simulink model "entryVehicle"  (R2025a)
settings: Solver=ode5  StartTime=startTime  StopTime=stopTime  FixedStep=stepTime  RelTol=1e-3
values from neighbouring files (symbols this model uses):
  alpha_0 = deg2rad(-23.)    [run_entryVehicle.m]
  alpha_T_CD = [0 5 10 15 20 25 30 35 40]    [ApolloDragCoeff.mat]
  alpha_T_CL = [0 5 10 15 20 25 30 35 40]    [ApolloLiftCoeff.mat]
  beta_0 = deg2rad(0.05)    [run_entryVehicle.m]
  CD_T = [1.13 1.305 1.34 1.394 1.445 1.472 1.48 1.468 1.454 1.486 1.51 1.124 ... (99 elements, 11x9)]    [ApolloDragCoeff.mat]
  chi_0 = deg2rad(90)    [run_entryVehicle.m]
  CL_T = [0 0 0 0 0 0 0 0 0 0 0 0.098 ... (99 elements, 11x9)]    [ApolloLiftCoeff.mat]
  d_ref = 3.9    [run_entryVehicle.m]
  gamma_0 = deg2rad(-9.536)    [run_entryVehicle.m]
  H_s = 7050    [run_entryVehicle.m]
  I_xx = 5617.61    [run_entryVehicle.m]
  I_xz = 0    [run_entryVehicle.m]
  I_yy = 4454.62    [run_entryVehicle.m]
  I_zz = 4454.80    (= 4454.8)    [run_entryVehicle.m]
  lambda_0 = deg2rad(0)    [run_entryVehicle.m]
  m_0 = 4976    [run_entryVehicle.m]
  Mach_numbers_CD = [0.9 1.1 1.2 1.35 1.65 2 2.4 3 4 6 10]    [ApolloDragCoeff.mat]
  Mach_numbers_CL = [0.9 1.1 1.2 1.35 1.65 2 2.4 3 4 6 10]    [ApolloLiftCoeff.mat]
  Mars_mu = 3.98319648e14    (= 398319648000000)    [run_entryVehicle.m]
  Mars_radius = 6371e3    (= 6371000)    [run_entryVehicle.m]
  p_0 = deg2rad(0)    [run_entryVehicle.m]
  q_0 = deg2rad(0)    [run_entryVehicle.m]
  r_0 = deg2rad(0)    [run_entryVehicle.m]
  R_0 = 220e3 + Mars_radius    (= 6591000)    [run_entryVehicle.m]
  r_cm = [1.57; 0; -0.137]    [run_entryVehicle.m]
  R_s = 287    [run_entryVehicle.m]
  rho_0 = 1.225    [run_entryVehicle.m]
  S_ref = 12    [run_entryVehicle.m]
  sigma_0 = deg2rad(110.)    [run_entryVehicle.m]
  specific_heat = 1.33    [run_entryVehicle.m]
  stepTime = 0.01    [run_entryVehicle.m]
  tau_0 = deg2rad(0)    [run_entryVehicle.m]
  V_0 = 11e3    (= 11000)    [run_entryVehicle.m]
undefined symbols (not defined in the file or in its folder): A_attitude, acce_bias, acce_S, alpha_T_Cm, alpha_T_Cm_q, B_attitude, Cm_qT, Cm_T, dynamics_constants, K_lat, K_long, lateral_ref, longitudinal_ref, Mach_numbers_Cm, Mach_numbers_Cm_q, my_max, Q0, r0_eci, rateGyro_bias, rateGyro_S, v0_eci
libraries: simulink_extras x32, simulink x3, SignalEditorBlockLib x1
(part 1 of 3)
settings Model: Creator=tester  LastModifiedBy=rafae

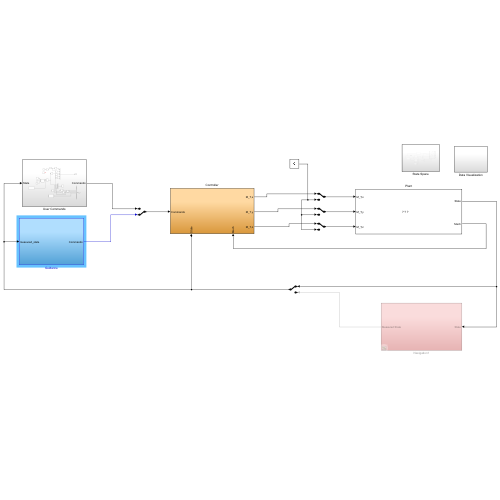
[thumbnail: Simulink's stored preview of the top-level diagram]
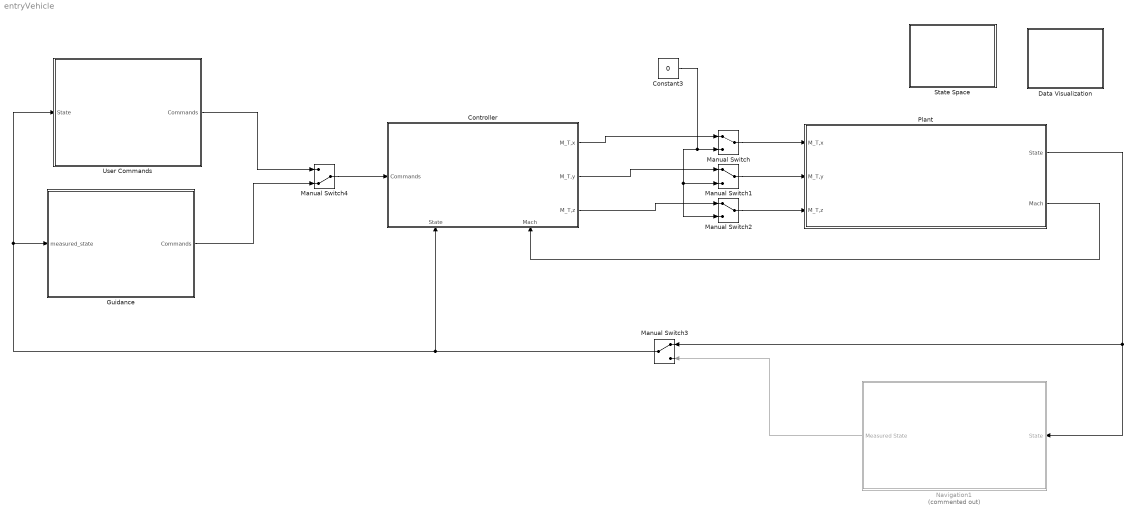
== system entryVehicle ==
  Constant3 : Constant  Value=0
  Controller : Subsystem
      settings: PortSchema="{\"entries\":[{\"content\":{\"sides\":[{\"content\":{\"connectorIds\":[\"In1\"]},\"type\":\"ConnectorPlacement.EquallySpacedRectSide\",\"uuid\":\"6730c763-0db7-4539-af59-842a5691e68e\"},{\"content\":{\"connectorIds\":[\"Out1\",\"Out2\",\"Out3\"],\"side\":\"RIGHT\"},\"type\":\"ConnectorPlacement.EquallySpacedRectSide\",\"uuid\":\"60c274f5-9a0e-4442-9031-a8a2f12bc615\"},{\"content\":{\"side\":\"TOP\"},\"type\":\"ConnectorPlacement.EquallySpacedRectSide\",\"uuid\":\"e1e9f683-9b0b-4096-8ce5-6b557ad43515\"},{\"content\":{\"connectorIds\":[\"In2\",\"In3\"],\"side\":\"BOTTOM\"},\"type\":\"ConnectorPlacement.EquallySpacedRectSide\",\"uuid\":\"b92da982-2d47-4e6b-9095-2c7c1889c431\"}]},\"type\":\"ConnectorPlacement.EquallySpacedConnector\",\"uuid\":\"278978b4-8d2f-4edc-bb2a-9785bc810a53\"}],\"packageUris\":[\"http://schema.mathworks.com/mf0/Connector/R2020b\"],\"version\":\"1.0\"}"
  Data Visualization : Subsystem
  Guidance : Subsystem
  Manual Switch{,1..3} (4 alike) : ManualSwitch
  Manual Switch4 : ManualSwitch  CurrentSetting=0
  Navigation1 : Subsystem  Commented=on
  Plant : Subsystem
      mask Display: image('MSLEntryVehicle.jpg', [0,0,0,0,100,90]);
  State Space : Subsystem
  User Commands : Subsystem
  wires:
  Controller/1(M_T,x) -> Manual Switch/1
  Manual Switch/1 -> Plant/1(M_T,x)
  Manual Switch2/1 -> Plant/3(M_T,z)
  Manual Switch1/1 -> Plant/2(M_T,y)
  Controller/2(M_T,y) -> Manual Switch1/1
  Controller/3(M_T,z) -> Manual Switch2/1
  Constant3/1 -> Manual Switch1/2, Manual Switch2/2, Manual Switch/2
  Plant/1(State) -> Navigation1/1(State), Manual Switch3/1
  Plant/2(Mach) -> Controller/3(Mach)
  User Commands/1(Commands) -> Manual Switch4/1
  Guidance/1(Commands) -> Manual Switch4/2
  Manual Switch4/1 -> Controller/1(Commands)
  Navigation1/1(Measured State) -> Manual Switch3/2
  Manual Switch3/1 -> Controller/2(State), User Commands/1(State), Guidance/1(measured_state)

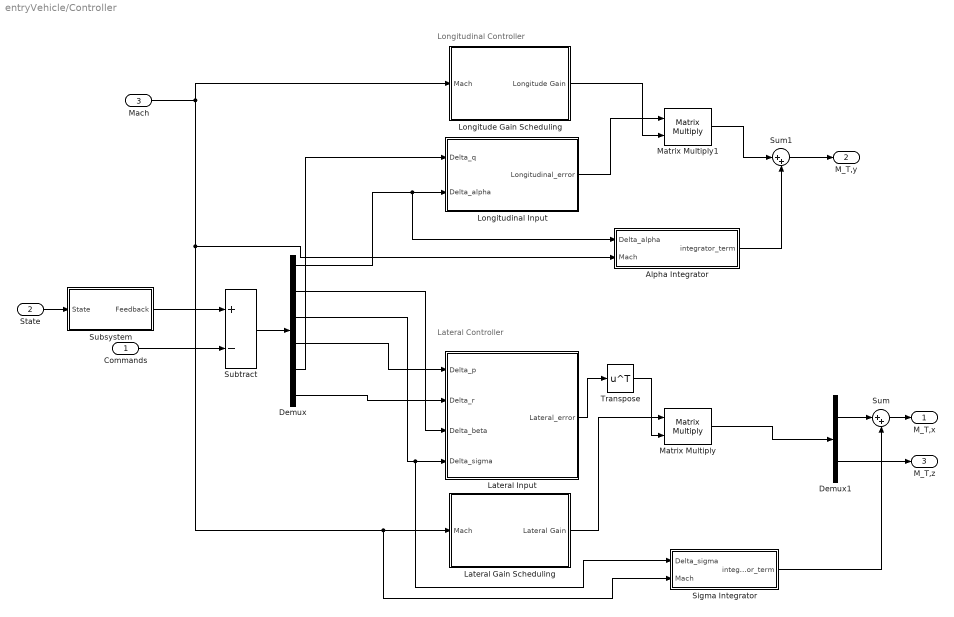
== system entryVehicle/Controller ==
  note: Lateral Controller
  note: Longitudinal Controller
  Commands : Inport
  State : Inport  Port=2
  Mach : Inport  Port=3
  Alpha Integrator : Subsystem
  Demux : Demux  Outputs=6
  Demux1 : Demux  Outputs=2
  Lateral Gain Scheduling : Subsystem
  Lateral Input : Subsystem
  Longitude Gain Scheduling : Subsystem
  Longitudinal Input : Subsystem
  Matrix Multiply : Product  Multiplication=Matrix(*)
  Matrix Multiply1 : Product  Multiplication=Matrix(*)
  Sigma Integrator : Subsystem
  Subsystem : Subsystem
  Subtract : Sum  Inputs=+-
  Sum : Sum  Inputs=|++
  Sum1 : Sum  Inputs=|++
  Transpose : Math  Operator=transpose
  M_T,x : Outport
  M_T,y : Outport  Port=2
  M_T,z : Outport  Port=3
  wires:
  State/1 -> Subsystem/1(State)
  Demux/1 -> Alpha Integrator/1(Delta_alpha), Longitudinal Input/2(Delta_alpha)
  Demux/5 -> Longitudinal Input/1(Delta_q)
  Demux/2 -> Lateral Input/3(Delta_beta)
  Demux/3 -> Lateral Input/4(Delta_sigma), Sigma Integrator/1(Delta_sigma)
  Demux/4 -> Lateral Input/1(Delta_p)
  Demux/6 -> Lateral Input/2(Delta_r)
  Commands/1 -> Subtract/2
  Subtract/1 -> Demux/1
  Subsystem/1(Feedback) -> Subtract/1
  Mach/1 -> Longitude Gain Scheduling/1(Mach), Alpha Integrator/2(Mach), Sigma Integrator/2(Mach), Lateral Gain Scheduling/1(Mach)
  Longitudinal Input/1(Longitudinal_error) -> Matrix Multiply1/1
  Longitude Gain Scheduling/1(Longitude Gain) -> Matrix Multiply1/2
  Matrix Multiply/1 -> Demux1/1
  Demux1/1 -> Sum/1
  Sum/1 -> M_T,x/1
  Matrix Multiply1/1 -> Sum1/1
  Sum1/1 -> M_T,y/1
  Demux1/2 -> M_T,z/1
  Lateral Gain Scheduling/1(Lateral Gain) -> Matrix Multiply/1
  Lateral Input/1(Lateral_error) -> Transpose/1
  Transpose/1 -> Matrix Multiply/2
  Alpha Integrator/1(integrator_term) -> Sum1/2
  Sigma Integrator/1(integrator_term) -> Sum/2

== system entryVehicle/Data Visualization ==

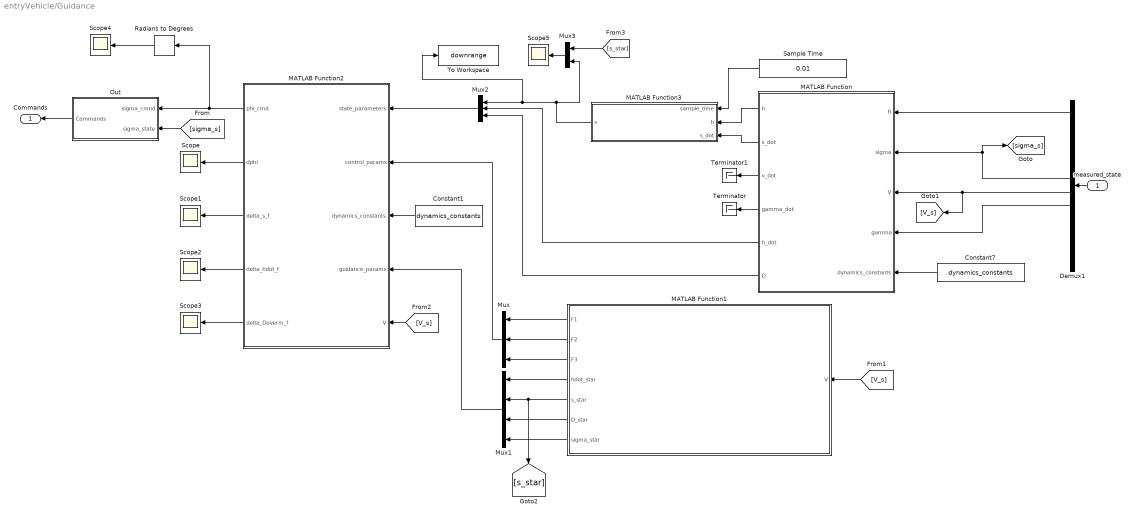
== system entryVehicle/Guidance ==
  measured_state : Inport
  Constant1 : Constant  Value=dynamics_constants
  Constant7 : Constant  Value=dynamics_constants
  Demux1 : Demux  Outputs=12
  MATLAB Function : MATLAB Function  TreatAsAtomicUnit=on
  MATLAB Function1 : MATLAB Function  TreatAsAtomicUnit=on
  MATLAB Function2 : MATLAB Function  TreatAsAtomicUnit=on  SystemSampleTime=1
  MATLAB Function3 : MATLAB Function  TreatAsAtomicUnit=on  SystemSampleTime=0.01
  Mux : Mux  Inputs=3
  Mux1 : Mux
  Mux2 : Mux  Inputs=3
  Mux3 : Mux  Inputs=2
  Out : Subsystem
  Radians to Degrees : simulink_extras/Transformations/Radians to Degrees
  Sample Time : Constant  Value=0.01
  Scope{,1..5} (6 alike) : Scope
      Scope settings: ActiveDisplayYMinimum=-0.02182  ActiveDisplayYMaximum=0.19635
      Scope1 settings: ActiveDisplayYMinimum=-5846.34757  ActiveDisplayYMaximum=52617.12815  DataLoggingVariableName=ScopeData2
      Scope2 settings: ActiveDisplayYMinimum=-1.55731  ActiveDisplayYMaximum=13.66679  DataLoggingVariableName=ScopeData3
      Scope3 settings: ActiveDisplayYMinimum=-781.36553  ActiveDisplayYMaximum=1579.10132  DataLoggingVariableName=ScopeData4
      Scope4 settings: ActiveDisplayYMinimum=4.375  ActiveDisplayYMaximum=110.625
      Scope5 settings: ActiveDisplayYMinimum=-224179.17494  ActiveDisplayYMaximum=2.01869737437E+6
  Terminator : Terminator
  Terminator1 : Terminator
  To Workspace : ToWorkspace  VariableName=downrange  SaveFormat=Structure With Time  SampleTime=-1
  Commands : Outport
  wires:
  measured_state/1 -> Demux1/1
  MATLAB Function/4(gamma_dot) -> Terminator/1
  Out/1(Commands) -> Commands/1
  Constant7/1 -> MATLAB Function/5(dynamics_constants)
  Demux1/1 -> MATLAB Function/1(R)
  Demux1/6 -> MATLAB Function/2(sigma), [sigma_s]
  Demux1/7 -> [V_s], MATLAB Function/3(V)
  Demux1/8 -> MATLAB Function/4(gamma)
  MATLAB Function/3(v_dot) -> Terminator1/1
  MATLAB Function/1(h) -> MATLAB Function3/2(h)
  MATLAB Function/2(s_dot) -> MATLAB Function3/3(s_dot)
  Sample Time/1 -> MATLAB Function3/1(sample_time)
  MATLAB Function1/1(F1) -> Mux/1
  MATLAB Function1/2(F2) -> Mux/2
  MATLAB Function1/3(F3) -> Mux/3
  MATLAB Function1/4(hdot_star) -> Mux1/1
  MATLAB Function1/5(s_star) -> Mux1/2, [s_star]
  MATLAB Function1/6(D_star) -> Mux1/3
  MATLAB Function1/7(sigma_star) -> Mux1/4
  MATLAB Function3/1(s) -> Mux3/2, Mux2/1, To Workspace/1
  MATLAB Function/5(h_dot) -> Mux2/2
  MATLAB Function/6(D) -> Mux2/3
  Mux2/1 -> MATLAB Function2/1(state_parameters)
  Mux/1 -> MATLAB Function2/2(control_params)
  Mux1/1 -> MATLAB Function2/4(guidance_params)
  Constant1/1 -> MATLAB Function2/3(dynamics_constants)
  MATLAB Function2/1(phi_cmd) -> Radians to Degrees/1, Out/1(sigma_cmnd)
  MATLAB Function2/2(dphi) -> Scope/1
  MATLAB Function2/3(delta_s_f) -> Scope1/1
  MATLAB Function2/4(delta_hdot_f) -> Scope2/1
  MATLAB Function2/5(delta_Doverm_f) -> Scope3/1
  Radians to Degrees/1 -> Scope4/1
  [sigma_s] -> Out/2(sigma_state)
  [V_s] -> MATLAB Function1/1(V)
  [V_s] -> MATLAB Function2/5(V)
  [s_star] -> Mux3/1
  Mux3/1 -> Scope5/1

== system entryVehicle/Navigation1 ==
  State : Inport
  Abs : Abs  SaturateOnIntegerOverflow=off
  Demux : Demux  Outputs=12
  Demux1 : Demux  Outputs=12
  Derivative : Derivative
  ECI State Propagation : Subsystem
  ECI State to State : Subsystem
  IMU Sensor : Subsystem
  MATLAB Function : MATLAB Function  TreatAsAtomicUnit=on
  Mux2 : Mux  Inputs=2
  Mux5 : Mux  Inputs=2
  Scope2 : Scope
      settings: ActiveDisplayYMinimum=-14.28055  ActiveDisplayYMaximum=128.52494  DataLoggingVariableName=ScopeData3
  Scope4 : Scope
      settings: ActiveDisplayYMinimum=-1.3626  ActiveDisplayYMaximum=0.15263  DataLoggingVariableName=ScopeData7
  State to Body (acce minus gravity) : Subsystem
  Measured State : Outport
  wires:
  State/1 -> Demux/1, State to Body (acce minus gravity)/1(state)
  ECI State to State/1(meas_state) -> Demux1/1, Measured State/1
  State to Body (acce minus gravity)/1(acce_body) -> IMU Sensor/1(acce_body), MATLAB Function/1(u)
  State to Body (acce minus gravity)/2(omega_body) -> IMU Sensor/2(omega_body)
  IMU Sensor/1(a_meas) -> ECI State Propagation/1(a_meas)
  IMU Sensor/2(omega_meas) -> ECI State Propagation/2(omega_meas)
  ECI State Propagation/1(meas_state_ECI) -> ECI State to State/1(meas_state_ECI)
  Abs/1 -> Mux2/1
  MATLAB Function/1(y) -> Mux2/2
  Mux2/1 -> Scope2/1
  Derivative/1 -> Abs/1
  Demux1/8 -> Mux5/2
  Mux5/1 -> Scope4/1
  Demux/7 -> Derivative/1
  State to Body (acce minus gravity)/3(Qtrue) -> ECI State Propagation/3(Q_true)
  Demux/8 -> Mux5/1

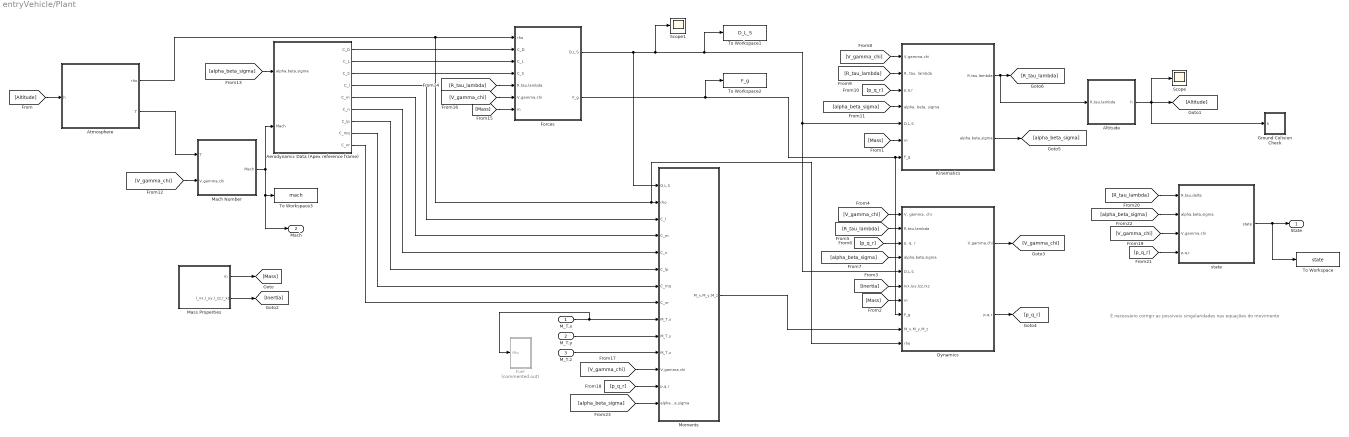
== system entryVehicle/Plant ==
  note: É necessário corrigir as possíveis singularidades nas equações do movimento
  M_T,x : Inport
  M_T,y : Inport  Port=2
  M_T,z : Inport  Port=3
  Aerodynamic Data (Apex reference frame) : Subsystem
  Altitude : Subsystem
  Atmosphere : Subsystem
  Dynamics : Subsystem
  Forces : Subsystem
  Fuel : Subsystem  Commented=on
  Ground Colision Check : Subsystem
  Kinematics : Subsystem
  Mach Number : Subsystem
  Mass Properties : Subsystem
  Moments : Subsystem
  Scope : Scope
      settings: ActiveDisplayYMinimum=-27500.49137  ActiveDisplayYMaximum=247500.0546  YLabel=m  DataLoggingVariableName=ScopeData7
  Scope1 : Scope
      settings: ActiveDisplayYMinimum=-224326.20631  ActiveDisplayYMaximum=477184.42934  DataLoggingVariableName=ScopeData2
  To Workspace : ToWorkspace  VariableName=state  SaveFormat=Structure With Time  SampleTime=-1
  To Workspace1 : ToWorkspace  VariableName=D_L_S  SaveFormat=Structure With Time  SampleTime=-1
  To Workspace2 : ToWorkspace  VariableName=F_g  SaveFormat=Structure With Time  SampleTime=-1
  To Workspace3 : ToWorkspace  VariableName=mach  SaveFormat=Structure With Time  SampleTime=-1
  state : Subsystem
  State : Outport
  Mach : Outport  Port=2
  wires:
  M_T,x/1 -> Fuel/1(Mtx), Moments/9(M_T,x)
  M_T,y/1 -> Moments/10(M_T,y)
  M_T,z/1 -> Moments/11(M_T,z)
  Aerodynamic Data (Apex reference frame)/6(C_n) -> Moments/5(C_n)
  Aerodynamic Data (Apex reference frame)/5(C_m) -> Moments/4(C_m)
  Aerodynamic Data (Apex reference frame)/4(C_l) -> Moments/3(C_l)
  Altitude/1(h) -> [Altitude], Scope/1, Ground Colision Check/1(h)
  [Altitude] -> Atmosphere/1(h)
  Mass Properties/1(m) -> [Mass]
  [Mass] -> Kinematics/6(m)
  Mass Properties/2(I_xx,I_yy,I_zz,I_xz) -> [Inertia]
  Forces/2(F_g) -> To Workspace2/1, Dynamics/8(F_g), Kinematics/7(F_g)
  [Mass] -> Dynamics/7(m)
  [Inertia] -> Dynamics/6(Ixx,Iyy,Izz,Ixz)
  Forces/1(D,L,S) -> Scope1/1, To Workspace1/1, Dynamics/5(D,L,S), Kinematics/5(D,L,S), Moments/1(D,L,S)
  Moments/1(M_x,M_y,M_z) -> Dynamics/9(M_x,M_y,M_z)
  Dynamics/2(p,q,r) -> [p_q_r]
  Dynamics/1(V,gamma,chi) -> [V_gamma_chi]
  Kinematics/2(alpha,beta,sigma) -> [alpha_beta_sigma]
  [V_gamma_chi] -> Dynamics/1("V, gamma, chi")
  [R_tau_lambda] -> Dynamics/2(R,tau,lambda)
  Kinematics/1(R,tau,lambda) -> [R_tau_lambda], Altitude/1(R,tau,lambda)
  [p_q_r] -> Dynamics/3("p, q, r")
  [alpha_beta_sigma] -> Dynamics/4(alpha,beta,sigma)
  [V_gamma_chi] -> Kinematics/1(V,gamma,chi)
  [R_tau_lambda] -> Kinematics/2("R, tau, lambda")
  [p_q_r] -> Kinematics/3(p,q,r)
  [alpha_beta_sigma] -> Kinematics/4("alpha, beta, sigma")
  Mach Number/1(Mach) -> To Workspace3/1, Mach/1, Aerodynamic Data (Apex reference frame)/2(Mach)
  [V_gamma_chi] -> Mach Number/2(V,gamma,chi)
  Atmosphere/1(rho) -> Dynamics/10(rho), Moments/2(rho), Forces/1(rho)
  [alpha_beta_sigma] -> Aerodynamic Data (Apex reference frame)/1(alpha,beta,sigma)
  [R_tau_lambda] -> Forces/5(R,tau,lambda)
  [Mass] -> Forces/7(m)
  [V_gamma_chi] -> Forces/6(V,gamma,chi)
  [V_gamma_chi] -> Moments/12(V,gamma,chi)
  Atmosphere/2(T) -> Mach Number/1(T)
  Aerodynamic Data (Apex reference frame)/1(C_D) -> Forces/2(C_D)
  Aerodynamic Data (Apex reference frame)/2(C_L) -> Forces/3(C_L)
  Aerodynamic Data (Apex reference frame)/3(C_S) -> Forces/4(C_S)
  [p_q_r] -> Moments/13(p,q,r)
  Aerodynamic Data (Apex reference frame)/9(C_nr) -> Moments/8(C_nr)
  Aerodynamic Data (Apex reference frame)/8(C_mq) -> Moments/7(C_mq)
  Aerodynamic Data (Apex reference frame)/7(C_lp) -> Moments/6(C_lp)
  [V_gamma_chi] -> state/3(V,gamma,chi)
  [R_tau_lambda] -> state/1(R,tau,delta)
  [p_q_r] -> state/4(p,q,r)
  [alpha_beta_sigma] -> state/2(alpha,beta,sigma)
  state/1(state) -> To Workspace/1, State/1
  [alpha_beta_sigma] -> Moments/14(alpha,beta,sigma)

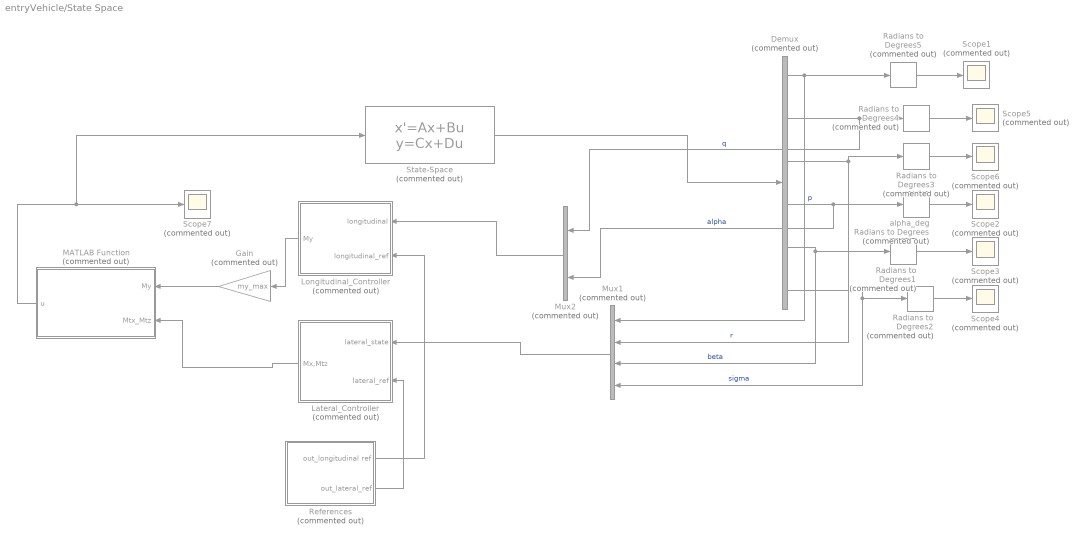
== system entryVehicle/State Space ==
  Demux : Demux  Commented=on  Outputs=6
  Gain : Gain  Commented=on  Gain=my_max
  Lateral_Controller : Subsystem  Commented=on
  Longitudinal_Controller : Subsystem  Commented=on
  MATLAB Function : MATLAB Function  Commented=on  TreatAsAtomicUnit=on
  Mux1 : Mux  Commented=on
  Mux2 : Mux  Commented=on  Inputs=2
  Radians to Degrees{1..5} (5 alike) : simulink_extras/Transformations/Radians to Degrees  Commented=on
  References : Subsystem  Commented=on
  Scope{1..7} (7 alike) : Scope  Commented=on
      Scope1 settings: ActiveDisplayYMinimum=-1.19941  ActiveDisplayYMaximum=0.17016
      Scope2 settings: ActiveDisplayYMinimum=-1.81589  ActiveDisplayYMaximum=2.88928  DataLoggingVariableName=ScopeData2
      Scope3 settings: ActiveDisplayYMinimum=-0.00061  ActiveDisplayYMaximum=0.00135
      Scope4 settings: ActiveDisplayYMinimum=-3.22061  ActiveDisplayYMaximum=28.98549  DataLoggingVariableName=ScopeData2
      Scope5 settings: ActiveDisplayYMinimum=-44.27214  ActiveDisplayYMaximum=39.05439  DataLoggingVariableName=ScopeData3
      Scope6 settings: ActiveDisplayYMinimum=-0.06363  ActiveDisplayYMaximum=0.53909  DataLoggingVariableName=ScopeData4
      Scope7 settings: ActiveDisplayYMinimum=-66691.93639  ActiveDisplayYMaximum=44857.66818  DataLoggingVariableName=ScopeData5
  State-Space : StateSpace  Commented=on  A=A_attitude  B=B_attitude  C=eye(6)  D=zeros(6,3)  InitialCondition=[0; 0; 0; -0.101; 0; 0]
  alpha_deg : simulink_extras/Transformations/Radians to Degrees  Commented=on
  wires:
  Radians to Degrees1/1 -> Scope3/1
  MATLAB Function/1(u) -> Scope7/1, State-Space/1
  Demux/4 -> alpha_deg/1, Mux2/2  "alpha"
  Radians to Degrees2/1 -> Scope4/1
  Lateral_Controller/1(Mx,Mtz) -> MATLAB Function/2(Mtx_Mtz)
  Demux/1 -> Mux1/1, Radians to Degrees5/1  "p"
  Longitudinal_Controller/1(My) -> Gain/1
  Demux/3 -> Mux1/2, Radians to Degrees3/1  "r"
  Demux/2 -> Mux2/1, Radians to Degrees4/1  "q"
  Demux/5 -> Mux1/3, Radians to Degrees1/1  "beta"
  Radians to Degrees3/1 -> Scope6/1
  Radians to Degrees5/1 -> Scope1/1
  Radians to Degrees4/1 -> Scope5/1
  Demux/6 -> Mux1/4, Radians to Degrees2/1  "sigma"
  State-Space/1 -> Demux/1
  alpha_deg/1 -> Scope2/1
  References/1(out_longitudinal ref) -> Longitudinal_Controller/2(longitudinal_ref)
  Mux1/1 -> Lateral_Controller/1(lateral_state)
  References/2(out_lateral_ref) -> Lateral_Controller/2(lateral_ref)
  Gain/1 -> MATLAB Function/1(My)
  Mux2/1 -> Longitudinal_Controller/1(longitudinal)

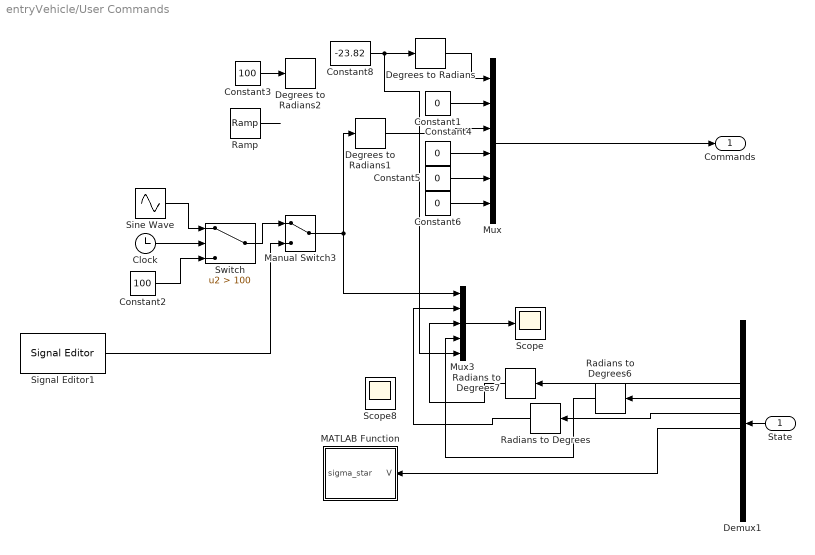
== system entryVehicle/User Commands ==
  State : Inport
  Clock : Clock
  Constant{1,4..6} (4 alike) : Constant  Value=0
  Constant2 : Constant  Value=100
  Constant3 : Constant  Value=100
  Constant8 : Constant  Value=-23.82
  Degrees to Radians : simulink_extras/Transformations/Degrees to Radians
  Degrees to Radians1 : simulink_extras/Transformations/Degrees to Radians
  Degrees to Radians2 : simulink_extras/Transformations/Degrees to Radians
  Demux1 : Demux  Outputs=12
  MATLAB Function : MATLAB Function  TreatAsAtomicUnit=on
  Manual Switch3 : ManualSwitch
  Mux : Mux  Inputs=6
  Mux3 : Mux  Inputs=5
  Radians to Degrees : simulink_extras/Transformations/Radians to Degrees
  Radians to Degrees6 : simulink_extras/Transformations/Radians to Degrees
  Radians to Degrees7 : simulink_extras/Transformations/Radians to Degrees
  Ramp : simulink/Sources/Ramp  slope=1  start=100  InitialOutput=70
  Scope : Scope
      settings: ActiveDisplayYMinimum=-42.06517  ActiveDisplayYMaximum=138.41018
  Scope8 : Scope
      settings: ActiveDisplayYMinimum=-1  ActiveDisplayYMaximum=1
  Signal Editor1 : SignalEditorBlockLib/Signal Editor  FileName=sigma_ref_dataset.mat  ActiveScenario=signalDataset  ActiveSignal=sigma_ref  IsBus=off  OutputBusObjectStr=Bus: BusObject  SampleTime=0  Interpolate=off  ZeroCross=off  OutputAfterFinalValue=Setting to zero  Unit=inherit  PreserveSignalName=on  ApplySigPropsToAllScenarios=on  ApplySigPropsToAllSignals=off
  Sine Wave : Sin  Amplitude=20  Bias=100  Frequency=0.05  Phase=1.2  SampleTime=0
  Switch : Switch  Criteria=u2 > Threshold  Threshold=100  SaturateOnIntegerOverflow=off  InputSameDT=off
  Commands : Outport
  wires:
  Radians to Degrees/1 -> Mux3/2
  Constant5/1 -> Mux/5
  Ramp/1 -> ?
  State/1 -> Demux1/1
  Constant4/1 -> Mux/4
  Sine Wave/1 -> Switch/1
  Constant6/1 -> Mux/6
  Demux1/5 -> Radians to Degrees6/1
  Radians to Degrees7/1 -> Mux3/3
  Constant2/1 -> Switch/3
  Degrees to Radians/1 -> Mux/1
  Mux/1 -> Commands/1
  Constant8/1 -> Mux3/5, Degrees to Radians/1
  Switch/1 -> Manual Switch3/1
  Manual Switch3/1 -> Mux3/1, Degrees to Radians1/1
  Mux3/1 -> Scope/1
  Demux1/4 -> Radians to Degrees7/1
  Demux1/6 -> Radians to Degrees/1
  Clock/1 -> Switch/2
  Constant1/1 -> Mux/2
  Radians to Degrees6/1 -> Mux3/4
  Demux1/7 -> MATLAB Function/1(V)
  Constant3/1 -> Degrees to Radians2/1
  Degrees to Radians1/1 -> Mux/3
  Signal Editor1/1 -> Manual Switch3/2

== system entryVehicle/Controller/Alpha Integrator ==
  Delta_alpha : Inport
  Mach : Inport  Port=2
  Gain1 : Gain  Gain=-1
  Gain2 : Gain  Gain=-1/100
  Integrator : Integrator
  MATLAB Function : MATLAB Function  TreatAsAtomicUnit=on
  Product : Product
  Scope : Scope
      settings: ActiveDisplayYMinimum=-61830.77216  ActiveDisplayYMaximum=555371.2989
  integrator_term : Outport
  wires:
  Delta_alpha/1 -> Integrator/1
  Mach/1 -> MATLAB Function/1(Mach)
  Integrator/1 -> Product/1
  MATLAB Function/1(K_integrator_alpha) -> Gain2/1, Scope/1
  Product/1 -> integrator_term/1
  Gain2/1 -> Product/2

== system entryVehicle/Controller/Lateral Gain Scheduling ==
  Mach : Inport
  Gain : Gain  Gain=-1
  MATLAB Function : MATLAB Function  TreatAsAtomicUnit=on
  Lateral Gain : Outport
  wires:
  Mach/1 -> MATLAB Function/1(Mach)
  Gain/1 -> Lateral Gain/1
  MATLAB Function/1(K_lat) -> Gain/1

== system entryVehicle/Controller/Lateral Input ==
  Delta_p : Inport
  Delta_r : Inport  Port=2
  Delta_beta : Inport  Port=3
  Delta_sigma : Inport  Port=4
  Mux : Mux
  Transpose : Math  Operator=transpose
  Lateral_error : Outport
  wires:
  Mux/1 -> Transpose/1
  Delta_r/1 -> Mux/2
  Delta_beta/1 -> Mux/3
  Transpose/1 -> Lateral_error/1
  Delta_p/1 -> Mux/1
  Delta_sigma/1 -> Mux/4

== system entryVehicle/Controller/Longitude Gain Scheduling ==
  Mach : Inport
  Gain : Gain  Gain=-1
  MATLAB Function : MATLAB Function  TreatAsAtomicUnit=on
  Longitude Gain : Outport
  wires:
  Mach/1 -> MATLAB Function/1(Mach)
  MATLAB Function/1(K_long) -> Gain/1
  Gain/1 -> Longitude Gain/1

== system entryVehicle/Controller/Longitudinal Input ==
  Delta_q : Inport
  Delta_alpha : Inport  Port=2
  Mux : Mux  Inputs=2
  Transpose1 : Math  Operator=transpose
  Longitudinal_error : Outport
  wires:
  Delta_q/1 -> Mux/1
  Delta_alpha/1 -> Mux/2
  Mux/1 -> Transpose1/1
  Transpose1/1 -> Longitudinal_error/1

== system entryVehicle/Controller/Sigma Integrator ==
  Delta_sigma : Inport
  Mach : Inport  Port=2
  Gain1 : Gain  Gain=1/100
  Gain2 : Gain
  Integrator : Integrator
  MATLAB Function : MATLAB Function  TreatAsAtomicUnit=on
  Product : Product
  Scope : Scope
      settings: ActiveDisplayYMinimum=-61830.77216  ActiveDisplayYMaximum=555371.2989
  integrator_term : Outport
  wires:
  Delta_sigma/1 -> Integrator/1
  Mach/1 -> MATLAB Function/1(Mach)
  Integrator/1 -> Product/1
  MATLAB Function/1(K_integrator_sigma) -> Gain1/1, Scope/1
  Product/1 -> integrator_term/1
  Gain1/1 -> Product/2

== system entryVehicle/Controller/Subsystem ==
  State : Inport
  Demux : Demux  Outputs=12
  Mux : Mux  Inputs=6
  Feedback : Outport
  wires:
  State/1 -> Demux/1
  Mux/1 -> Feedback/1
  Demux/4 -> Mux/1  "alpha"
  Demux/5 -> Mux/2  "beta"
  Demux/6 -> Mux/3  "sigma"
  Demux/10 -> Mux/4  "p"
  Demux/12 -> Mux/6  "r"
  Demux/11 -> Mux/5  "q"

== system entryVehicle/Guidance/Out ==
  sigma_cmnd : Inport
  sigma_state : Inport  Port=2
  Constant{7,9..11} (4 alike) : Constant  Value=0
  Constant8 : Constant  Value=-23.82
  Degrees to Radians : simulink_extras/Transformations/Degrees to Radians
  Mux : Mux  Inputs=2
  Mux3 : Mux  Inputs=6
  Radians to Degrees : simulink_extras/Transformations/Radians to Degrees
  Scope : Scope
      settings: ActiveDisplayYMinimum=1.32812  ActiveDisplayYMaximum=136.03251  DataLoggingVariableName=ScopeData3
  Commands : Outport
  wires:
  Constant7/1 -> Mux3/2
  Constant11/1 -> Mux3/6
  Mux3/1 -> Commands/1
  Constant8/1 -> Degrees to Radians/1
  Constant10/1 -> Mux3/5
  Degrees to Radians/1 -> Mux3/1
  Constant9/1 -> Mux3/4
  sigma_cmnd/1 -> Mux/1, Mux3/3
  sigma_state/1 -> Mux/2
  Mux/1 -> Radians to Degrees/1
  Radians to Degrees/1 -> Scope/1

== system entryVehicle/Navigation1/ECI State Propagation ==
  note: Inertial Position Propagation
  note: Inertial Velocity Propagation
  note: Intertial Attitude Propagation
  a_meas : Inport
  omega_meas : Inport  Port=2
  Q_true : Inport  Port=3
  Constant : Constant  Value=Mars_mu
  Integrator3 : Integrator  InitialCondition=Q0
  Integrator4 : Integrator  InitialCondition=v0_eci
  Integrator5 : Integrator  InitialCondition=r0_eci
  MATLAB Function : MATLAB Function  TreatAsAtomicUnit=on
  MATLAB Function1 : MATLAB Function  TreatAsAtomicUnit=on
  MATLAB Function2 : MATLAB Function  TreatAsAtomicUnit=on
  MATLAB Function3 : MATLAB Function  TreatAsAtomicUnit=on
  Mux : Mux
  Product1 : Product  Multiplication=Matrix(*)
  Scope : Scope
      settings: DataLoggingVariableName=ScopeData10
  Sum1 : Sum  Inputs=|++
  meas_state_ECI : Outport
  wires:
  omega_meas/1 -> MATLAB Function2/2(omega), Mux/4  "omega_meas"
  Integrator3/1 -> MATLAB Function/1(Q_in)
  MATLAB Function1/1(TIC) -> Product1/1
  a_meas/1 -> Product1/2
  Product1/1 -> Sum1/1
  Sum1/1 -> Integrator4/1
  Integrator4/1 -> Mux/2, Integrator5/1  "v_meas_ECI"
  Integrator5/1 -> MATLAB Function3/1(r_ECI), Mux/1  "r_meas_ECI"
  Mux/1 -> meas_state_ECI/1
  MATLAB Function3/1(g_vec_ECI) -> Scope/1, Sum1/2
  Constant/1 -> MATLAB Function3/2(mu)
  MATLAB Function2/1(Q_dot) -> Integrator3/1
  MATLAB Function/1(Q_out) -> MATLAB Function2/1(Q)  "Q_meas_ECI"
  Q_true/1 -> Mux/3, MATLAB Function1/1(Q)

== system entryVehicle/Navigation1/ECI State to State ==
  meas_state_ECI : Inport
  V_gamma_chi : Inport  Port=2
  R_tau_delta : Inport  Port=3
  Demux : Demux  Outputs=13
  MATLAB Function : MATLAB Function  TreatAsAtomicUnit=on
  MATLAB Function1 : MATLAB Function  TreatAsAtomicUnit=on
  MATLAB Function3 : MATLAB Function  TreatAsAtomicUnit=on
  Mux : Mux  Inputs=3
  Mux1 : Mux  Inputs=3
  Mux2 : Mux
  Mux3 : Mux  Inputs=3
  Mux4 : Mux
  meas_state : Outport
  wires:
  meas_state_ECI/1 -> Demux/1
  Demux/2 -> Mux/2  "r_y"
  Demux/6 -> Mux1/3  "v_z"
  Demux/5 -> Mux1/2  "v_y"
  Demux/3 -> Mux/3  "r_z"
  Demux/1 -> Mux/1  "r_x"
  Demux/4 -> Mux1/1  "v_x"
  Demux/7 -> Mux2/1  "q1"
  Demux/8 -> Mux2/2  "q2"
  Demux/9 -> Mux2/3  "q3"
  Demux/10 -> Mux2/4  "q4"
  Mux/1 -> MATLAB Function/1(r_ECI)  "r_ECI"
  Mux1/1 -> MATLAB Function1/1(v_ECI)  "v_ECI"
  Mux2/1 -> MATLAB Function3/1(Q)  "Q"
  MATLAB Function1/1(V_gamma_chi) -> MATLAB Function3/2(V_gamma_chi), Mux4/3
  MATLAB Function/1(R_tau_delta) -> MATLAB Function3/3(R_tau_delta), MATLAB Function1/2(R_tau_delta), Mux4/1
  Demux/13 -> Mux3/3  "r"
  Demux/11 -> Mux3/1  "p"
  Demux/12 -> Mux3/2  "q"
  Mux4/1 -> meas_state/1
  MATLAB Function3/1(alpha_beta_sigma) -> Mux4/2
  Mux3/1 -> Mux4/4  "p_q_r"

== system entryVehicle/Navigation1/IMU Sensor ==
  note: Rate Gyroscopes
  note: Accelerometers
  acce_body : Inport
  omega_body : Inport  Port=2
  Accelerometer Sensor Noise : simulink/Sources/Band-Limited White Noise  Cov=[0.1]  Ts=stepTime  seed=[23341]
  Constant : Constant  Value=acce_bias
  Constant1 : Constant  Value=acce_S
  Constant2 : Constant  Value=rateGyro_bias
  Constant3 : Constant  Value=rateGyro_S
  Constant4 : Constant  Value=0
  Constant5 : Constant  Value=0
  MATLAB Function : MATLAB Function  TreatAsAtomicUnit=on
  MATLAB Function1 : MATLAB Function  TreatAsAtomicUnit=on
  Manual Switch : ManualSwitch
  Manual Switch1 : ManualSwitch
  Rate Gyro Sensor Noise : simulink/Sources/Band-Limited White Noise  Cov=[0.1]  Ts=stepTime  seed=[23341]
  Sum : Sum  Inputs=|++
  Sum1 : Sum  Inputs=|++
  a_meas : Outport
  omega_meas : Outport  Port=2
  wires:
  Constant/1 -> MATLAB Function/2(b_a)
  acce_body/1 -> MATLAB Function/1(a_body)
  Constant1/1 -> MATLAB Function/3(S_a)
  omega_body/1 -> MATLAB Function1/1(omega_true)
  Constant3/1 -> MATLAB Function1/3(S_omega)
  Constant2/1 -> MATLAB Function1/2(b_gyro)
  MATLAB Function/1(a_measured) -> Sum/1
  Sum/1 -> a_meas/1
  MATLAB Function1/1(omega_measured) -> Sum1/1
  Sum1/1 -> omega_meas/1
  Manual Switch/1 -> Sum/2
  Accelerometer Sensor Noise/1 -> Manual Switch/2
  Constant4/1 -> Manual Switch/1
  Constant5/1 -> Manual Switch1/1
  Manual Switch1/1 -> Sum1/2
  Rate Gyro Sensor Noise/1 -> Manual Switch1/2

== system entryVehicle/Navigation1/State to Body (acce minus gravity) ==
  state : Inport
  Constant : Constant  Value=Mars_mu
  Demux2 : Demux  Outputs=12
  Derivative1 : Derivative
  MATLAB Function : MATLAB Function  TreatAsAtomicUnit=on
  MATLAB Function1 : MATLAB Function  TreatAsAtomicUnit=on
  MATLAB Function2 : MATLAB Function  TreatAsAtomicUnit=on
  MATLAB Function3 : MATLAB Function  TreatAsAtomicUnit=on
  MATLAB Function4 : MATLAB Function  Commented=on  TreatAsAtomicUnit=on
  MATLAB Function5 : MATLAB Function  TreatAsAtomicUnit=on
  Mux{2,4..6} (4 alike) : Mux  Inputs=3
  Scope : Scope
      settings: ActiveDisplayYMinimum=-108.94936  ActiveDisplayYMaximum=93.01266
  Subtract : Sum  Inputs=+-
  acce_body : Outport
  omega_body : Outport  Port=2
  Qtrue : Outport  Port=3
  R_tau_delta : Outport  Port=4
  V_gamma_chi : Outport  Port=5
  wires:
  state/1 -> Demux2/1
  Demux2/10 -> Mux4/1  "p"
  Demux2/11 -> Mux4/2  "q"
  Demux2/12 -> Mux4/3  "r"
  Demux2/7 -> Mux5/1  "V"
  Demux2/8 -> Mux5/2  "gamma"
  Demux2/9 -> Mux5/3  "chi"
  Demux2/4 -> Mux6/1  "alpha"
  Demux2/5 -> Mux6/2  "beta"
  Demux2/6 -> Mux6/3  "sigma"
  Mux4/1 -> omega_body/1  "omega"
  Mux5/1 -> MATLAB Function/3(V_gamma_chi), V_gamma_chi/1, MATLAB Function3/2(V_gamma_chi), MATLAB Function5/2(V_gamma_chi), MATLAB Function2/1(V_gamma_chi)  "V_gamma_chi"
  Mux6/1 -> MATLAB Function5/4(alpha_beta_sigma), MATLAB Function3/1(alpha_beta_sigma), MATLAB Function/1(alpha_beta_sigma)  "alpha_beta_sigma"
  Subtract/1 -> acce_body/1, Scope/1
  Demux2/2 -> Mux2/2
  Demux2/3 -> Mux2/3
  Derivative1/1 -> MATLAB Function5/1(acce_ECI)  "acce_ECI"
  MATLAB Function3/1(g_b) -> Subtract/2
  Constant/1 -> MATLAB Function3/4(mu)
  Demux2/1 -> Mux2/1
  Mux2/1 -> MATLAB Function2/2(R_tau_delta), MATLAB Function5/3(R_tau_delta), MATLAB Function3/3(R_tau_delta), MATLAB Function/2(R_tau_delta), R_tau_delta/1  "R_tau_delta"
  MATLAB Function/1(Qtrue) -> Qtrue/1
  MATLAB Function2/1(V_ECI) -> Derivative1/1
  MATLAB Function5/1(acce_body) -> Subtract/1

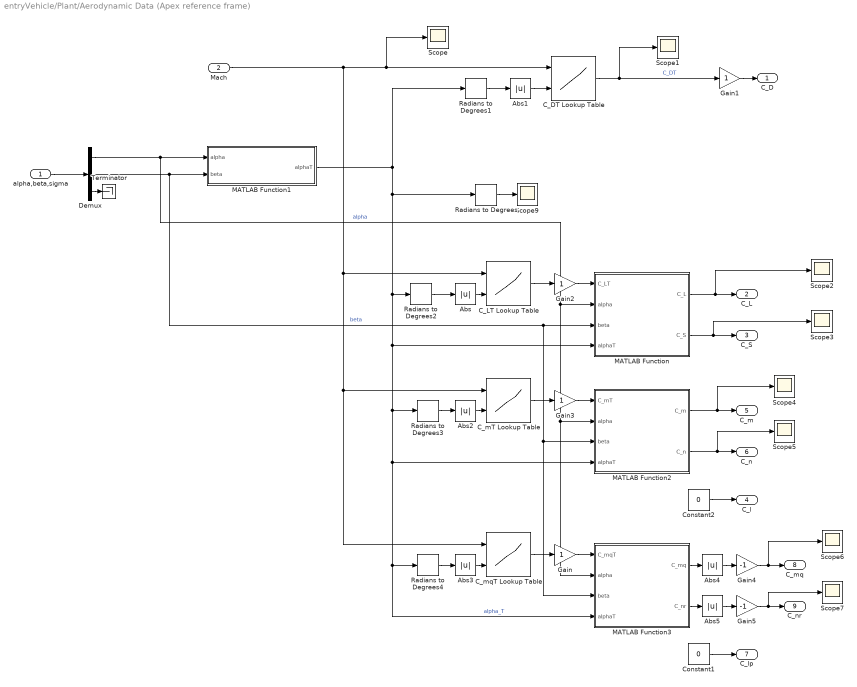
== system entryVehicle/Plant/Aerodynamic Data (Apex reference frame) ==
  alpha,beta,sigma : Inport
  Mach : Inport  Port=2
  Abs{,1..5} (6 alike) : Abs  SaturateOnIntegerOverflow=off
  C_DT Lookup Table : Lookup_n-D  BreakpointsForDimension1=Mach_numbers_CD  BreakpointsForDimension2=alpha_T_CD  Table=CD_T  ExtrapMethod=Clip  InternalRulePriority=Speed  RndMeth=Simplest
      settings: InputPortMap=u0,u1
  C_LT Lookup Table : Lookup_n-D  BreakpointsForDimension1=Mach_numbers_CL  BreakpointsForDimension2=alpha_T_CL  Table=CL_T  ExtrapMethod=Clip  InternalRulePriority=Speed  RndMeth=Simplest
      settings: InputPortMap=u0,u1
  C_mT Lookup Table : Lookup_n-D  BreakpointsForDimension1=Mach_numbers_Cm  BreakpointsForDimension2=alpha_T_Cm  Table=Cm_T  ExtrapMethod=Clip  InternalRulePriority=Speed  RndMeth=Simplest
      settings: InputPortMap=u0,u1
  C_mqT Lookup Table : Lookup_n-D  BreakpointsForDimension1=Mach_numbers_Cm_q  BreakpointsForDimension2=alpha_T_Cm_q  Table=Cm_qT  ExtrapMethod=Clip  InternalRulePriority=Speed  RndMeth=Simplest
      settings: InputPortMap=u0,u1
  Constant1 : Constant  Value=0  SampleTime=stepTime
  Constant2 : Constant  Value=0  SampleTime=stepTime
  Demux : Demux  Outputs=3
  Gain{,1..3} (4 alike) : Gain
  Gain4 : Gain  Gain=-1
  Gain5 : Gain  Gain=-1
  MATLAB Function : MATLAB Function  TreatAsAtomicUnit=on
  MATLAB Function1 : MATLAB Function  TreatAsAtomicUnit=on
  MATLAB Function2 : MATLAB Function  TreatAsAtomicUnit=on
  MATLAB Function3 : MATLAB Function  TreatAsAtomicUnit=on
  Radians to Degrees{,1..4} (5 alike) : simulink_extras/Transformations/Radians to Degrees
  Scope{,1..7,9} (9 alike) : Scope
      Scope settings: ActiveDisplayYMinimum=-3.97377  ActiveDisplayYMaximum=38.23182
      Scope1 settings: ActiveDisplayYMinimum=1.21884  ActiveDisplayYMaximum=1.22011
      Scope2 settings: ActiveDisplayYMinimum=-0.53017  ActiveDisplayYMaximum=-0.38679
      Scope3 settings: ActiveDisplayYMinimum=-0.04806  ActiveDisplayYMaximum=0.02843  DataLoggingVariableName=ScopeData2
      Scope4 settings: ActiveDisplayYMinimum=0.32825  ActiveDisplayYMaximum=0.41118  DataLoggingVariableName=ScopeData5
      Scope5 settings: ActiveDisplayYMinimum=-0.0399  ActiveDisplayYMaximum=0.02225  DataLoggingVariableName=ScopeData6
      Scope6 settings: ActiveDisplayYMinimum=-1.19833  ActiveDisplayYMaximum=-0.30954  DataLoggingVariableName=ScopeData7
      Scope7 settings: ActiveDisplayYMinimum=-1  ActiveDisplayYMaximum=1  DataLoggingVariableName=ScopeData8
      Scope9 settings: ActiveDisplayYMinimum=23.55985  ActiveDisplayYMaximum=32.96181
  Terminator : Terminator
  C_D : Outport
  C_L : Outport  Port=2
  C_S : Outport  Port=3
  C_l : Outport  Port=4
  C_m : Outport  Port=5
  C_n : Outport  Port=6
  C_lp : Outport  Port=7
  C_mq : Outport  Port=8
  C_nr : Outport  Port=9
  wires:
  alpha,beta,sigma/1 -> Demux/1
  Demux/1 -> MATLAB Function1/1(alpha), MATLAB Function3/2(alpha), MATLAB Function2/2(alpha), MATLAB Function/2(alpha)  "alpha"
  Demux/2 -> MATLAB Function1/2(beta), MATLAB Function/3(beta), MATLAB Function3/3(beta), MATLAB Function2/3(beta)  "beta"
  Demux/3 -> Terminator/1
  Constant2/1 -> C_l/1
  MATLAB Function1/1(alphaT) -> Radians to Degrees1/1, Radians to Degrees/1, Radians to Degrees2/1, MATLAB Function/4(alphaT), Radians to Degrees3/1, MATLAB Function2/4(alphaT), Radians to Degrees4/1, MATLAB Function3/4(alphaT)  "alpha_T"
  C_DT Lookup Table/1 -> Gain1/1, Scope1/1  "C_DT"
  MATLAB Function/1(C_L) -> Scope2/1, C_L/1
  MATLAB Function/2(C_S) -> Scope3/1, C_S/1
  C_mT Lookup Table/1 -> Gain3/1
  MATLAB Function2/1(C_m) -> C_m/1, Scope4/1
  MATLAB Function2/2(C_n) -> Scope5/1, C_n/1
  MATLAB Function3/2(C_nr) -> Abs5/1
  MATLAB Function3/1(C_mq) -> Abs4/1
  Constant1/1 -> C_lp/1
  Abs/1 -> C_LT Lookup Table/2
  Abs1/1 -> C_DT Lookup Table/2
  Abs3/1 -> C_mqT Lookup Table/2
  Abs2/1 -> C_mT Lookup Table/2
  Radians to Degrees/1 -> Scope9/1
  Radians to Degrees1/1 -> Abs1/1
  Radians to Degrees2/1 -> Abs/1
  Radians to Degrees3/1 -> Abs2/1
  Radians to Degrees4/1 -> Abs3/1
  C_LT Lookup Table/1 -> Gain2/1
  Mach/1 -> Scope/1, C_DT Lookup Table/1, C_mqT Lookup Table/1, C_mT Lookup Table/1, C_LT Lookup Table/1
  C_mqT Lookup Table/1 -> Gain/1
  Gain/1 -> MATLAB Function3/1(C_mqT)
  Gain1/1 -> C_D/1
  Gain2/1 -> MATLAB Function/1(C_LT)
  Gain3/1 -> MATLAB Function2/1(C_mT)
  Abs4/1 -> Gain4/1
  Gain4/1 -> C_mq/1, Scope6/1
  Abs5/1 -> Gain5/1
  Gain5/1 -> C_nr/1, Scope7/1

== system entryVehicle/Plant/Altitude ==
  R,tau,lambda : Inport
  Constant : Constant  Value=Mars_radius  SampleTime=stepTime
  Demux : Demux  Outputs=3
  Sum : Sum  Inputs=|+-
  Terminator : Terminator
  Terminator1 : Terminator
  h : Outport
  wires:
  Constant/1 -> Sum/2
  Sum/1 -> h/1
  Demux/1 -> Sum/1  "R"
  R,tau,lambda/1 -> Demux/1
  Demux/2 -> Terminator/1
  Demux/3 -> Terminator1/1

== system entryVehicle/Plant/Atmosphere ==
  h : Inport
  Atmospheric Density : Subsystem
  Constant : Constant  Value=288  SampleTime=stepTime
  Scope : Scope
      settings: ActiveDisplayYMinimum=-0.15314  ActiveDisplayYMaximum=1.37825  YLabel=kg/m^3  DataLoggingVariableName=ScopeData10
  To Workspace : ToWorkspace  VariableName=rho  SaveFormat=Structure With Time  SampleTime=-1
  rho : Outport
  T : Outport  Port=2
  wires:
  h/1 -> Atmospheric Density/1(h)
  Atmospheric Density/1(rho) -> To Workspace/1, Scope/1, rho/1
  Constant/1 -> T/1

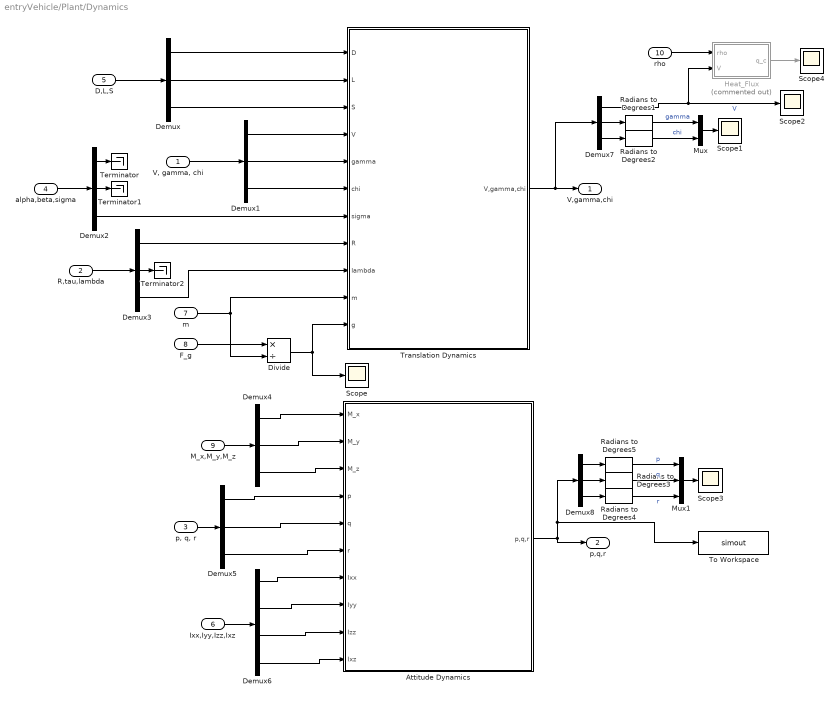
== system entryVehicle/Plant/Dynamics ==
  "V, gamma, chi" : Inport
  R,tau,lambda : Inport  Port=2
  "p, q, r" : Inport  Port=3
  alpha,beta,sigma : Inport  Port=4
  D,L,S : Inport  Port=5
  Ixx,Iyy,Izz,Ixz : Inport  Port=6
  m : Inport  Port=7
  F_g : Inport  Port=8
  M_x,M_y,M_z : Inport  Port=9
  rho : Inport  Port=10
  Attitude Dynamics : Subsystem
  Demux{,1..5,7..8} (8 alike) : Demux  Outputs=3
  Demux6 : Demux
  Divide : Product  Inputs=*/
  Heat_Flux : Subsystem  Commented=on
  Mux : Mux  Inputs=2
  Mux1 : Mux  Inputs=3
  Radians to Degrees{1..5} (5 alike) : simulink_extras/Transformations/Radians to Degrees
  Scope{,1..4} (5 alike) : Scope
      Scope settings: ActiveDisplayYMinimum=9.08863  ActiveDisplayYMaximum=9.89386
      Scope1 settings: ActiveDisplayYMinimum=-661.88299  ActiveDisplayYMaximum=372.33186  YLabel=deg
      Scope2 settings: ActiveDisplayYMinimum=-1297.16838  ActiveDisplayYMaximum=12484.04868  YLabel=m/s  DataLoggingVariableName=ScopeData5
      Scope3 settings: ActiveDisplayYMinimum=-3.08802  ActiveDisplayYMaximum=2.99348  YLabel=deg/s  DataLoggingVariableName=ScopeData6
      Scope4 settings: ActiveDisplayYMinimum=-1  ActiveDisplayYMaximum=1
  Terminator : Terminator
  Terminator1 : Terminator
  Terminator2 : Terminator
  To Workspace : ToWorkspace  VariableName=simout  SaveFormat=Structure With Time  SampleTime=-1
  Translation Dynamics : Subsystem
  V,gamma,chi : Outport
  p,q,r : Outport  Port=2
  wires:
  Translation Dynamics/1(V,gamma,chi) -> Demux7/1, V,gamma,chi/1
  Attitude Dynamics/1(p,q,r) -> p,q,r/1, Demux8/1, To Workspace/1
  Demux/2 -> Translation Dynamics/2(L)
  Demux/1 -> Translation Dynamics/1(D)
  Demux/3 -> Translation Dynamics/3(S)
  D,L,S/1 -> Demux/1
  "V, gamma, chi"/1 -> Demux1/1
  Demux1/1 -> Translation Dynamics/4(V)
  Demux1/2 -> Translation Dynamics/5(gamma)
  Demux1/3 -> Translation Dynamics/6(chi)
  alpha,beta,sigma/1 -> Demux2/1
  Demux2/3 -> Translation Dynamics/7(sigma)
  Demux2/1 -> Terminator/1
  Demux2/2 -> Terminator1/1
  R,tau,lambda/1 -> Demux3/1
  Demux3/1 -> Translation Dynamics/8(R)
  Demux3/3 -> Translation Dynamics/9(lambda)
  Demux3/2 -> Terminator2/1
  Demux4/2 -> Attitude Dynamics/2(M_y)
  Demux4/1 -> Attitude Dynamics/1(M_x)
  Demux4/3 -> Attitude Dynamics/3(M_z)
  M_x,M_y,M_z/1 -> Demux4/1
  "p, q, r"/1 -> Demux5/1
  Demux5/1 -> Attitude Dynamics/4(p)
  Demux5/2 -> Attitude Dynamics/5(q)
  Demux5/3 -> Attitude Dynamics/6(r)
  Demux6/1 -> Attitude Dynamics/7(Ixx)
  Demux6/2 -> Attitude Dynamics/8(Iyy)
  Demux6/3 -> Attitude Dynamics/9(Izz)
  Ixx,Iyy,Izz,Ixz/1 -> Demux6/1
  Demux6/4 -> Attitude Dynamics/10(Ixz)
  m/1 -> Divide/2, Translation Dynamics/10(m)
  Divide/1 -> Scope/1, Translation Dynamics/11(g)
  F_g/1 -> Divide/1
  Radians to Degrees4/1 -> Mux1/3  "r"
  Demux8/2 -> Radians to Degrees3/1
  Demux8/1 -> Radians to Degrees5/1
  Mux1/1 -> Scope3/1
  Radians to Degrees3/1 -> Mux1/2  "q"
  Radians to Degrees5/1 -> Mux1/1  "p"
  Demux8/3 -> Radians to Degrees4/1
  Radians to Degrees2/1 -> Mux/2  "chi"
  Demux7/3 -> Radians to Degrees2/1
  Demux7/1 -> Heat_Flux/2(V), Scope2/1  "V"
  Demux7/2 -> Radians to Degrees1/1
  Radians to Degrees1/1 -> Mux/1  "gamma"
  Mux/1 -> Scope1/1
  rho/1 -> Heat_Flux/1(rho)
  Heat_Flux/1(q_c) -> Scope4/1

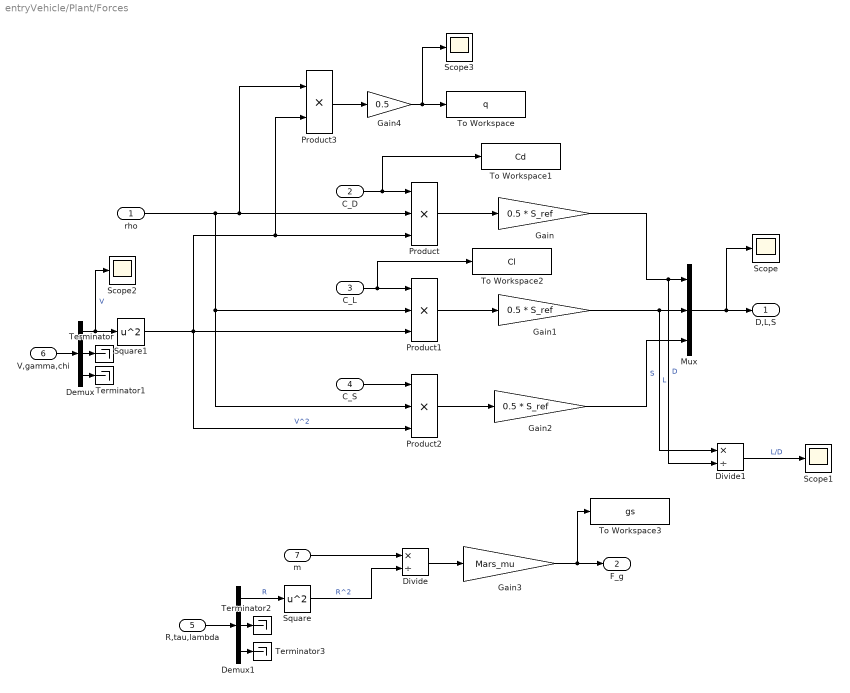
== system entryVehicle/Plant/Forces ==
  rho : Inport
  C_D : Inport  Port=2
  C_L : Inport  Port=3
  C_S : Inport  Port=4
  R,tau,lambda : Inport  Port=5
  V,gamma,chi : Inport  Port=6
  m : Inport  Port=7
  Demux : Demux  Outputs=3
  Demux1 : Demux  Outputs=3
  Divide : Product  Inputs=*/
  Divide1 : Product  Inputs=*/
  Gain : Gain  Gain=0.5 * S_ref
  Gain1 : Gain  Gain=0.5 * S_ref
  Gain2 : Gain  Gain=0.5 * S_ref
  Gain3 : Gain  Gain=Mars_mu
  Gain4 : Gain  Gain=0.5
  Mux : Mux  Inputs=3
  Product : Product  Inputs=3
  Product1 : Product  Inputs=3
  Product2 : Product  Inputs=3
  Product3 : Product
  Scope{,1..3} (4 alike) : Scope
      Scope settings: SampleTime=stepTime  ActiveDisplayYMinimum=-518882.36321  ActiveDisplayYMaximum=1.10386890877E+6  DataLoggingVariableName=ScopeData3
      Scope1 settings: ActiveDisplayYMinimum=-0.38738  ActiveDisplayYMaximum=-0.36454
      Scope2 settings: ActiveDisplayYMinimum=3510.4145  ActiveDisplayYMaximum=5776.34624  DataLoggingVariableName=ScopeData4
      Scope3 settings: ActiveDisplayYMinimum=-4679.56934  ActiveDisplayYMaximum=42116.12406  DataLoggingVariableName=ScopeData8
  Square : Math  Operator=square  OutputSignalType=real
  Square1 : Math  Operator=square
  Terminator{,1..3} (4 alike) : Terminator
  To Workspace : ToWorkspace  VariableName=q  SaveFormat=Structure With Time  SampleTime=-1
  To Workspace1 : ToWorkspace  VariableName=Cd  SaveFormat=Structure With Time  SampleTime=-1
  To Workspace2 : ToWorkspace  VariableName=Cl  SaveFormat=Structure With Time  SampleTime=-1
  To Workspace3 : ToWorkspace  VariableName=gs  SaveFormat=Structure With Time  SampleTime=-1
  D,L,S : Outport
  F_g : Outport  Port=2
  wires:
  C_D/1 -> To Workspace1/1, Product/1
  rho/1 -> Product2/2, Product1/2, Product/2, Product3/1
  V,gamma,chi/1 -> Demux/1
  Demux/2 -> Terminator/1
  Demux/3 -> Terminator1/1
  Product/1 -> Gain/1
  C_L/1 -> To Workspace2/1, Product1/1
  C_S/1 -> Product2/1
  Product1/1 -> Gain1/1
  Product2/1 -> Gain2/1
  Gain1/1 -> Divide1/1, Mux/2  "L"
  Gain/1 -> Mux/1, Divide1/2  "D"
  Gain2/1 -> Mux/3  "S"
  Mux/1 -> D,L,S/1, Scope/1
  Demux1/2 -> Terminator2/1
  Demux1/3 -> Terminator3/1
  R,tau,lambda/1 -> Demux1/1
  m/1 -> Divide/1
  Divide/1 -> Gain3/1
  Gain3/1 -> To Workspace3/1, F_g/1
  Demux1/1 -> Square/1  "R"
  Square/1 -> Divide/2  "R^2"
  Demux/1 -> Scope2/1, Square1/1  "V"
  Square1/1 -> Product2/3, Product/3, Product3/2, Product1/3  "V^2"
  Divide1/1 -> Scope1/1  "L/D"
  Product3/1 -> Gain4/1
  Gain4/1 -> To Workspace/1, Scope3/1

== system entryVehicle/Plant/Fuel ==
  Mtx : Inport
  Impulse : Scope
      settings: ActiveDisplayYMinimum=-210606.73617  ActiveDisplayYMaximum=1.89544194841E+6
  Integrator : Integrator
  To Workspace4 : ToWorkspace  VariableName=impulse  SaveFormat=Timeseries  SampleTime=-1
  wires:
  Integrator/1 -> To Workspace4/1, Impulse/1
  Mtx/1 -> Integrator/1

== system entryVehicle/Plant/Ground Colision Check ==
  h : Inport
  Constant : Constant  Value=0  SampleTime=stepTime
  Constant1 : Constant  SampleTime=stepTime
  Stop Simulation : Stop
  Switch : Switch  SaturateOnIntegerOverflow=off  InputSameDT=off
  wires:
  Switch/1 -> Stop Simulation/1
  Constant/1 -> Switch/1
  Constant1/1 -> Switch/3
  h/1 -> Switch/2

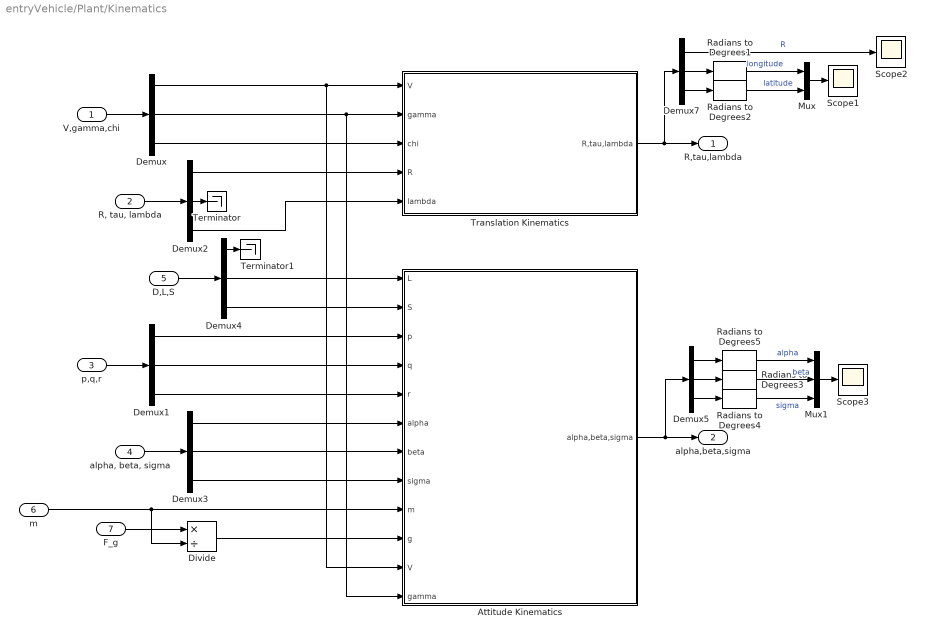
== system entryVehicle/Plant/Kinematics ==
  V,gamma,chi : Inport
  "R, tau, lambda" : Inport  Port=2
  p,q,r : Inport  Port=3
  "alpha, beta, sigma" : Inport  Port=4
  D,L,S : Inport  Port=5
  m : Inport  Port=6
  F_g : Inport  Port=7
  Attitude Kinematics : Subsystem
  Demux{,1..5,7} (7 alike) : Demux  Outputs=3
  Divide : Product  Inputs=*/
  Mux : Mux  Inputs=2
  Mux1 : Mux  Inputs=3
  Radians to Degrees{1..5} (5 alike) : simulink_extras/Transformations/Radians to Degrees
  Scope1 : Scope
      settings: ActiveDisplayYMinimum=-2.42277  ActiveDisplayYMaximum=17.48655  YLabel=deg  DataLoggingVariableName=ScopeData8
  Scope2 : Scope
      settings: ActiveDisplayYMinimum=6.34349950863E+6  ActiveDisplayYMaximum=6.6185000546E+6  YLabel=m  DataLoggingVariableName=ScopeData9
  Scope3 : Scope
      settings: ActiveDisplayYMinimum=-224.99897  ActiveDisplayYMaximum=224.99969  YLabel=deg  DataLoggingVariableName=ScopeData2
  Terminator : Terminator
  Terminator1 : Terminator
  Translation Kinematics : Subsystem
  R,tau,lambda : Outport
  alpha,beta,sigma : Outport  Port=2
  wires:
  Translation Kinematics/1(R,tau,lambda) -> Demux7/1, R,tau,lambda/1
  Attitude Kinematics/1(alpha,beta,sigma) -> Demux5/1, alpha,beta,sigma/1
  V,gamma,chi/1 -> Demux/1
  Demux/1 -> Translation Kinematics/1(V), Attitude Kinematics/11(V)
  Demux/2 -> Attitude Kinematics/12(gamma), Translation Kinematics/2(gamma)
  Demux/3 -> Translation Kinematics/3(chi)
  p,q,r/1 -> Demux1/1
  Demux1/1 -> Attitude Kinematics/3(p)
  Demux1/2 -> Attitude Kinematics/4(q)
  Demux1/3 -> Attitude Kinematics/5(r)
  "R, tau, lambda"/1 -> Demux2/1
  Demux2/1 -> Translation Kinematics/4(R)
  Demux2/3 -> Translation Kinematics/5(lambda)
  Demux3/2 -> Attitude Kinematics/7(beta)
  Demux3/1 -> Attitude Kinematics/6(alpha)
  Demux3/3 -> Attitude Kinematics/8(sigma)
  "alpha, beta, sigma"/1 -> Demux3/1
  m/1 -> Divide/2, Attitude Kinematics/9(m)
  Divide/1 -> Attitude Kinematics/10(g)
  F_g/1 -> Divide/1
  Demux2/2 -> Terminator/1
  D,L,S/1 -> Demux4/1
  Demux4/2 -> Attitude Kinematics/1(L)
  Demux4/3 -> Attitude Kinematics/2(S)
  Demux4/1 -> Terminator1/1
  Mux/1 -> Scope1/1
  Demux7/1 -> Scope2/1  "R"
  Demux7/2 -> Radians to Degrees1/1
  Demux7/3 -> Radians to Degrees2/1
  Radians to Degrees2/1 -> Mux/2  "latitude"
  Radians to Degrees1/1 -> Mux/1  "longitude"
  Radians to Degrees4/1 -> Mux1/3  "sigma"
  Demux5/3 -> Radians to Degrees4/1
  Demux5/2 -> Radians to Degrees3/1
  Radians to Degrees3/1 -> Mux1/2  "beta"
  Mux1/1 -> Scope3/1
  Demux5/1 -> Radians to Degrees5/1
  Radians to Degrees5/1 -> Mux1/1  "alpha"

== system entryVehicle/Plant/Mach Number ==
  T : Inport
  V,gamma,chi : Inport  Port=2
  Constant : Constant  Value=5
  Demux : Demux  Outputs=3
  Divide : Product  Inputs=*/
  Gain : Gain  Gain=specific_heat * R_s
  Manual Switch : ManualSwitch  CurrentSetting=0
  Scope : Scope
      settings: ActiveDisplayYMinimum=226.53674  ActiveDisplayYMaximum=426.53674  DataLoggingVariableName=ScopeData10
  Scope1 : Scope
      settings: ActiveDisplayYMinimum=-3.9725  ActiveDisplayYMaximum=38.23168
  Square Root : Sqrt  OutputSignalType=real
  Terminator : Terminator
  Terminator1 : Terminator
  Mach : Outport
  wires:
  V,gamma,chi/1 -> Demux/1
  Demux/3 -> Terminator/1
  Demux/2 -> Terminator1/1
  Demux/1 -> Divide/1  "V"
  Square Root/1 -> Scope/1, Divide/2  "a"
  T/1 -> Gain/1
  Gain/1 -> Square Root/1
  Divide/1 -> Manual Switch/2
  Manual Switch/1 -> Scope1/1, Mach/1
  Constant/1 -> Manual Switch/1

== system entryVehicle/Plant/Mass Properties ==
  Constant : Constant  Value=m_0  SampleTime=stepTime
  Constant1 : Constant  Value=I_xx  SampleTime=stepTime
  Constant2 : Constant  Value=I_yy  SampleTime=stepTime
  Constant3 : Constant  Value=I_zz  SampleTime=stepTime
  Constant4 : Constant  Value=I_xz  SampleTime=stepTime
  Mux : Mux
  m : Outport
  I_xx,I_yy,I_zz,I_xz : Outport  Port=2
  wires:
  Constant/1 -> m/1
  Constant2/1 -> Mux/2
  Constant3/1 -> Mux/3
  Constant1/1 -> Mux/1
  Constant4/1 -> Mux/4
  Mux/1 -> I_xx,I_yy,I_zz,I_xz/1

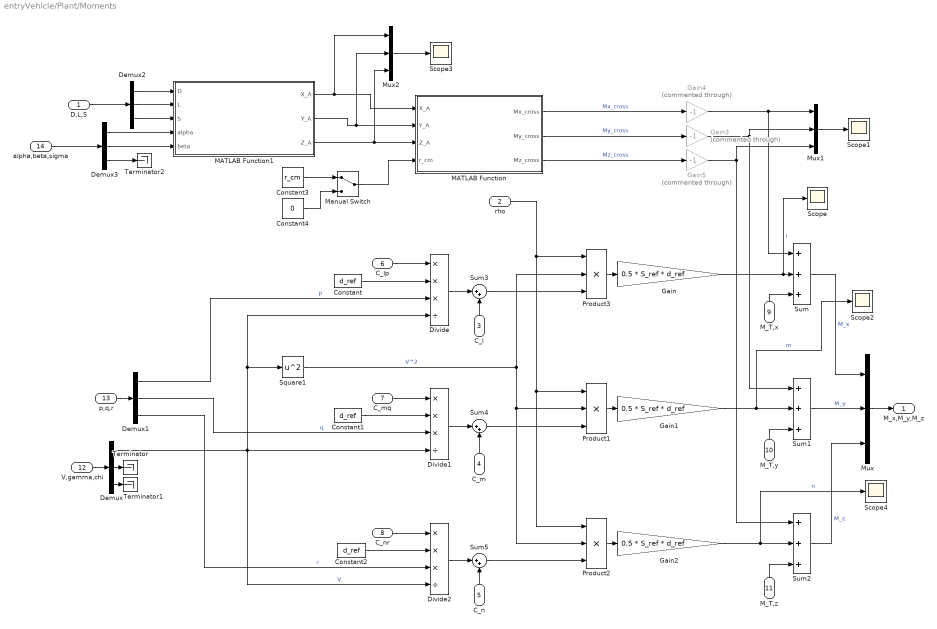
== system entryVehicle/Plant/Moments ==
  D,L,S : Inport
  rho : Inport  Port=2
  C_l : Inport  Port=3
  C_m : Inport  Port=4
  C_n : Inport  Port=5
  C_lp : Inport  Port=6
  C_mq : Inport  Port=7
  C_nr : Inport  Port=8
  M_T,x : Inport  Port=9
  M_T,y : Inport  Port=10
  M_T,z : Inport  Port=11
  V,gamma,chi : Inport  Port=12
  p,q,r : Inport  Port=13
  alpha,beta,sigma : Inport  Port=14
  Constant : Constant  Value=d_ref  SampleTime=stepTime
  Constant1 : Constant  Value=d_ref  SampleTime=stepTime
  Constant2 : Constant  Value=d_ref  SampleTime=stepTime
  Constant3 : Constant  Value=r_cm
  Constant4 : Constant  Value=0
  Demux{,1..3} (4 alike) : Demux  Outputs=3
  Divide : Product  Inputs=***/
  Divide1 : Product  Inputs=***/
  Divide2 : Product  Inputs=***/
  Gain : Gain  Gain=0.5 * S_ref * d_ref
  Gain1 : Gain  Gain=0.5 * S_ref * d_ref
  Gain2 : Gain  Gain=0.5 * S_ref * d_ref
  Gain3 : Gain  Commented=through  Gain=-1
  Gain4 : Gain  Commented=through  Gain=-1
  Gain5 : Gain  Commented=through  Gain=-1
  MATLAB Function : MATLAB Function  TreatAsAtomicUnit=on
  MATLAB Function1 : MATLAB Function  TreatAsAtomicUnit=on
  Manual Switch : ManualSwitch
  Mux : Mux  Inputs=3
  Mux1 : Mux  Inputs=3
  Mux2 : Mux  Inputs=3
  Product1 : Product  Inputs=3
  Product2 : Product  Inputs=3
  Product3 : Product  Inputs=3
  Scope{,1..4} (5 alike) : Scope
      Scope1 settings: ActiveDisplayYMinimum=-1.34461502134E+6  ActiveDisplayYMaximum=153349.65939  DataLoggingVariableName=ScopeData2
      Scope2 settings: ActiveDisplayYMinimum=-77022.88398  ActiveDisplayYMaximum=693205.95625  DataLoggingVariableName=ScopeData2
      Scope3 settings: DataLoggingVariableName=ScopeData4
      Scope4 settings: ActiveDisplayYMinimum=-3232.48131  ActiveDisplayYMaximum=3231.82766  DataLoggingVariableName=ScopeData3
  Square1 : Math  Operator=square
  Sum : Sum  Inputs=+|+|+
  Sum1 : Sum  Inputs=+|+|+
  Sum2 : Sum  Inputs=+|+|+
  Sum3 : Sum  Inputs=|++
  Sum4 : Sum  Inputs=|++
  Sum5 : Sum  Inputs=|++
  Terminator : Terminator
  Terminator1 : Terminator
  Terminator2 : Terminator
  M_x,M_y,M_z : Outport
  wires:
  Gain2/1 -> Scope4/1, Sum2/2  "n"
  V,gamma,chi/1 -> Demux/1
  Gain1/1 -> Scope2/1, Sum1/2  "m"
  Gain/1 -> Scope/1, Sum/2  "l"
  Demux/3 -> Terminator1/1
  Demux/1 -> Divide2/4, Divide1/4, Divide/4, Square1/1  "V"
  Product1/1 -> Gain1/1
  Demux/2 -> Terminator/1
  Product2/1 -> Gain2/1
  M_T,x/1 -> Sum/3
  M_T,y/1 -> Sum1/3
  M_T,z/1 -> Sum2/3
  Sum1/1 -> Mux/2  "M_y"
  Sum/1 -> Mux/1  "M_x"
  Sum2/1 -> Mux/3  "M_z"
  Mux/1 -> M_x,M_y,M_z/1
  p,q,r/1 -> Demux1/1
  Product3/1 -> Gain/1
  C_l/1 -> Sum3/2
  C_lp/1 -> Divide/1
  Demux1/1 -> Divide/3  "p"
  Sum3/1 -> Product3/3
  Divide/1 -> Sum3/1
  Constant/1 -> Divide/2
  rho/1 -> Product3/1, Product2/1, Product1/1
  Divide1/1 -> Sum4/1
  Sum4/1 -> Product1/3
  C_m/1 -> Sum4/2
  Divide2/1 -> Sum5/1
  Sum5/1 -> Product2/3
  C_n/1 -> Sum5/2
  C_mq/1 -> Divide1/1
  C_nr/1 -> Divide2/1
  Constant1/1 -> Divide1/2
  Constant2/1 -> Divide2/2
  Square1/1 -> Product2/2, Product1/2, Product3/2  "V^2"
  Demux1/2 -> Divide1/3  "q"
  Demux1/3 -> Divide2/3  "r"
  D,L,S/1 -> Demux2/1
  Manual Switch/1 -> MATLAB Function/4(r_cm)
  MATLAB Function/1(Mx_cross) -> Gain4/1  "Mx_cross"
  MATLAB Function/2(My_cross) -> Gain3/1  "My_cross"
  MATLAB Function/3(Mz_cross) -> Gain5/1  "Mz_cross"
  Constant3/1 -> Manual Switch/1
  Constant4/1 -> Manual Switch/2
  Demux2/1 -> MATLAB Function1/1(D)
  Demux2/2 -> MATLAB Function1/2(L)
  Demux2/3 -> MATLAB Function1/3(S)
  Demux3/1 -> MATLAB Function1/4(alpha)
  Demux3/2 -> MATLAB Function1/5(beta)
  alpha,beta,sigma/1 -> Demux3/1
  Demux3/3 -> Terminator2/1
  MATLAB Function1/1(X_A) -> MATLAB Function/1(X_A), Mux2/1
  MATLAB Function1/2(Y_A) -> MATLAB Function/2(Y_A), Mux2/2
  MATLAB Function1/3(Z_A) -> Mux2/3, MATLAB Function/3(Z_A)
  Mux1/1 -> Scope1/1
  Mux2/1 -> Scope3/1
  Gain3/1 -> Mux1/2, Sum1/1
  Gain4/1 -> Mux1/1, Sum/1
  Gain5/1 -> Mux1/3, Sum2/1

== system entryVehicle/Plant/state ==
  R,tau,delta : Inport
  alpha,beta,sigma : Inport  Port=2
  V,gamma,chi : Inport  Port=3
  p,q,r : Inport  Port=4
  Mux : Mux
  state : Outport
  wires:
  Mux/1 -> state/1
  R,tau,delta/1 -> Mux/1
  alpha,beta,sigma/1 -> Mux/2
  V,gamma,chi/1 -> Mux/3
  p,q,r/1 -> Mux/4
